simulink model "PD_Direct_Drive"  (R2016b)
settings: Solver=FixedStepAuto  StartTime=0.0  StopTime=inf  RelTol=1e-3  EnableMultiTasking=on
undefined symbols (not defined in the file): RGBLED_COLOR_ENUM, RGBLED_MODE_ENUM
libraries: pixhawk_slib_sensors_actuators x7, pixhawk_slib_misc_utils x6, simulink x2
settings Model: Creator=juanc  LastModifiedBy=pixhawk
settings OptimizationCC: DefaultParameterBehavior=Inlined  InlineInvariantSignals=on  LifeSpan=1  MaxStackSize=64
settings DebuggingCC: SFUnexpectedBacktrackingDiag=warning  SFNoUnconditionalDefaultTransitionDiag=warning  SFExecutionAtInitializationDiag=none
settings HardwareCC: ProdBitPerPointer=32  ProdBitPerSizeT=32  ProdBitPerPtrDiffT=32  ProdLargestAtomicInteger=Long  ProdLargestAtomicFloat=Double  ProdWordSize=32  ProdHWDeviceType=ARM Compatible->ARM Cortex
settings RTWCC: SystemTargetFile=ert.tlc  HardwareBoard=Pixhawk PX4  TLCOptions=-aInlineSetEventsForThisBaseRateFcn=TLC_FALSE -aSuppressMultiTaskScheduler=TLC_FALSE -aRateBasedStepFcn=0  TemplateMakefile=ert_default_tmf  Description=Embedded Coder  GenerateReport=on  Toolchain=Pixhawk Toolchain  IncludeHyperlinkInReport=on  LaunchReport=on  GenerateTraceInfo=on  GenerateTraceReport=on  GenerateTraceReportSl=on  GenerateTraceReportSf=on  GenerateTraceReportEml=on
settings CodeAppCC: ForceParamTrailComments=on  IgnoreCustomStorageClasses=off  OperatorAnnotations=on  SimulinkDataObjDesc=on  SFDataObjDesc=on  MATLABFcnDesc=on  InsertBlockDesc=on  MATLABSourceComments=on
settings ERTTargetCC: InlinedParameterPlacement=NonHierarchical  ERTCustomFileTemplate=PX4_codertarget_file_process.tlc
settings ConfigComp: CovMetricSettings=dw  CovHtmlReporting=on  CovSaveCumulativeToWorkspaceVar=on  CovSaveSingleToWorkspaceVar=on  CovExternalEMLEnable=off

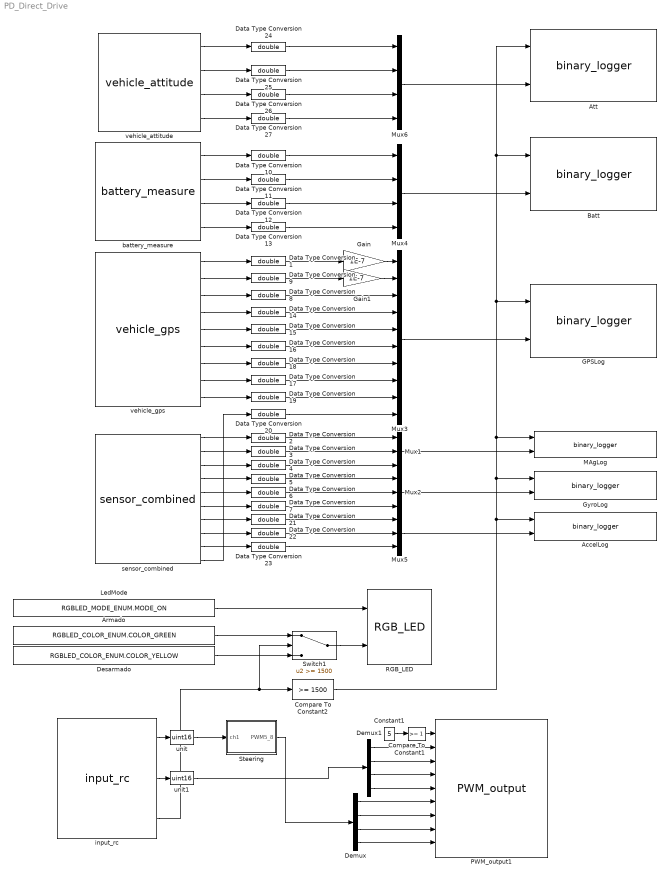
== system PD_Direct_Drive ==
  AccelLog : pixhawk_slib_misc_utils/binary_logger  logfile=/fs/microsd/log/acc  cacheflag=off  numRecs=1000
  Armado : Constant  Value=RGBLED_COLOR_ENUM.COLOR_GREEN  OutDataTypeStr=Enum: RGBLED_COLOR_ENUM
  Att : pixhawk_slib_misc_utils/binary_logger  logfile=/fs/microsd/log/att  cacheflag=off  numRecs=1000
  Batt : pixhawk_slib_misc_utils/binary_logger  logfile=/fs/microsd/log/bat  cacheflag=off  numRecs=1000
  Compare To Constant1 : simulink/Logic and Bit Operations/Compare To Constant  relop=>=  const=1  OutDataTypeStr=boolean
  Compare To Constant2 : simulink/Logic and Bit Operations/Compare To Constant  relop=>=  const=1500  OutDataTypeStr=boolean
  Constant1 : Constant  Value=5  OutDataTypeStr=Inherit: Inherit via back propagation  SampleTime=0.004
  Data Type Conversion{1..27} (27 alike) : DataTypeConversion  OutDataTypeStr=double
  Demux : Demux
  Demux1 : Demux
  Desarmado : Constant  Value=RGBLED_COLOR_ENUM.COLOR_YELLOW  OutDataTypeStr=Enum: RGBLED_COLOR_ENUM
  GPSLog : pixhawk_slib_misc_utils/binary_logger  logfile=/fs/microsd/log/GPS  cacheflag=off  numRecs=1000
  Gain : Gain  Gain=1E-7
  Gain1 : Gain  Gain=1E-7
  GyroLog : pixhawk_slib_misc_utils/binary_logger  logfile=/fs/microsd/log/gyr  cacheflag=off  numRecs=1000
  LedMode : Constant  Value=RGBLED_MODE_ENUM.MODE_ON  OutDataTypeStr=Enum: RGBLED_MODE_ENUM
  MAgLog : pixhawk_slib_misc_utils/binary_logger  logfile=/fs/microsd/log/mag  cacheflag=off  numRecs=1000
  Mux1 : Mux  Inputs=3
  Mux2 : Mux  Inputs=3
  Mux3 : Mux  Inputs=10
  Mux4 : Mux
  Mux5 : Mux  Inputs=3
  Mux6 : Mux
  PWM_output1 : pixhawk_slib_sensors_actuators/PWM_output  pwm_rate=50Hz  show_pwm1=on  show_pwm2=on  show_pwm3=on  show_pwm4=on  show_pwm5=on  show_pwm6=on  show_pwm7=on  show_pwm8=on
  RGB_LED : pixhawk_slib_sensors_actuators/RGB_LED
  Steering : MATLAB Function  TreatAsAtomicUnit=on
  Switch1 : Switch  Threshold=1500
  battery_measure : pixhawk_slib_sensors_actuators/battery_measure  SampleTime=1/250  VoltageOut=on  VoltageFilteredOut=off  CurrentOut=on  mAH_Out=on  TimeStamp=on
  input_rc : pixhawk_slib_sensors_actuators/input_rc  sampletime=1/250  channel1=on  channel2=off  channel3=on  channel4=off  channel5=off  channel6=off  channel7=on  channel8=off  ch_count=off  rssi=off  rc_failsafe=off  rc_lost=off  rc_inputsource=off
  sensor_combined : pixhawk_slib_sensors_actuators/sensor_combined  sampletime=1/250  show_mag=on  show_acc=on  show_gyro=on  show_baro=off  show_ts=on
  unit : DataTypeConversion  OutDataTypeStr=uint16
  unit1 : DataTypeConversion  OutDataTypeStr=uint16
  vehicle_attitude : pixhawk_slib_sensors_actuators/vehicle_attitude  sampletime=1/250  show_r=on  show_p=on  show_y=on  show_q=on
  vehicle_gps : pixhawk_slib_sensors_actuators/vehicle_gps  sampletime=1/250  show_ts_pos=on  show_alt=on  show_ts_gps=on  show_vel=on  show_fixtype=on  show_numsat=on
  wires:
  Switch1/1 -> RGB_LED/2
  Armado/1 -> Switch1/1
  Desarmado/1 -> Switch1/3
  LedMode/1 -> RGB_LED/1
  Data Type Conversion2/1 -> Mux1/1
  Data Type Conversion3/1 -> Mux1/2
  Data Type Conversion4/1 -> Mux1/3
  sensor_combined/2 -> Data Type Conversion3/1
  sensor_combined/3 -> Data Type Conversion4/1
  Mux2/1 -> GyroLog/2
  Data Type Conversion5/1 -> Mux2/1
  Data Type Conversion6/1 -> Mux2/2
  Data Type Conversion7/1 -> Mux2/3
  sensor_combined/1 -> Data Type Conversion2/1
  sensor_combined/4 -> Data Type Conversion5/1
  sensor_combined/5 -> Data Type Conversion6/1
  input_rc/3 -> Compare To Constant2/1, Switch1/2
  Mux3/1 -> GPSLog/2
  Compare To Constant2/1 -> Batt/1, Att/1, GPSLog/1, MAgLog/1, GyroLog/1, AccelLog/1
  Data Type Conversion1/1 -> Gain/1
  Data Type Conversion9/1 -> Gain1/1
  Data Type Conversion8/1 -> Mux3/3
  vehicle_gps/2 -> Data Type Conversion9/1
  vehicle_gps/3 -> Data Type Conversion8/1
  vehicle_gps/1 -> Data Type Conversion1/1
  vehicle_gps/4 -> Data Type Conversion14/1
  vehicle_gps/5 -> Data Type Conversion15/1
  vehicle_gps/9 -> Data Type Conversion19/1
  vehicle_gps/8 -> Data Type Conversion17/1
  vehicle_gps/7 -> Data Type Conversion18/1
  vehicle_gps/6 -> Data Type Conversion16/1
  battery_measure/4 -> Data Type Conversion13/1
  battery_measure/3 -> Data Type Conversion12/1
  battery_measure/1 -> Data Type Conversion10/1
  battery_measure/2 -> Data Type Conversion11/1
  Mux4/1 -> Batt/2
  Data Type Conversion10/1 -> Mux4/1
  Data Type Conversion11/1 -> Mux4/2
  Data Type Conversion12/1 -> Mux4/3
  Data Type Conversion14/1 -> Mux3/4
  Data Type Conversion15/1 -> Mux3/5
  Data Type Conversion13/1 -> Mux4/4
  Data Type Conversion16/1 -> Mux3/6
  Data Type Conversion17/1 -> Mux3/8
  Data Type Conversion18/1 -> Mux3/7
  Data Type Conversion19/1 -> Mux3/9
  Mux1/1 -> MAgLog/2
  Mux5/1 -> AccelLog/2
  Data Type Conversion21/1 -> Mux5/1
  Data Type Conversion22/1 -> Mux5/2
  Data Type Conversion23/1 -> Mux5/3
  sensor_combined/6 -> Data Type Conversion7/1
  sensor_combined/8 -> Data Type Conversion22/1
  sensor_combined/10 -> Data Type Conversion20/1
  Data Type Conversion20/1 -> Mux3/10
  vehicle_attitude/4 -> Data Type Conversion27/1
  vehicle_attitude/3 -> Data Type Conversion26/1
  vehicle_attitude/1 -> Data Type Conversion24/1
  vehicle_attitude/2 -> Data Type Conversion25/1
  Mux6/1 -> Att/2
  Data Type Conversion24/1 -> Mux6/1
  Data Type Conversion25/1 -> Mux6/2
  Data Type Conversion26/1 -> Mux6/3
  Data Type Conversion27/1 -> Mux6/4
  sensor_combined/7 -> Data Type Conversion21/1
  sensor_combined/9 -> Data Type Conversion23/1
  Gain/1 -> Mux3/1
  Gain1/1 -> Mux3/2
  Constant1/1 -> Compare To Constant1/1
  Compare To Constant1/1 -> PWM_output1/1
  input_rc/1 -> unit/1
  input_rc/2 -> unit1/1
  Demux/1 -> PWM_output1/6
  Demux/2 -> PWM_output1/7
  Demux/3 -> PWM_output1/8
  Demux/4 -> PWM_output1/9
  Steering/1(PWM5_8) -> Demux/1
  unit/1 -> Steering/1(ch1)
  Demux1/2 -> PWM_output1/3
  Demux1/3 -> PWM_output1/4
  Demux1/4 -> PWM_output1/5
  Demux1/1 -> PWM_output1/2
  unit1/1 -> Demux1/1

== matlab function PD_Direct_Drive/Steering ==
  data: ch1 input; PWM5_8 output
function PWM5_8 = fcn(ch1)
ang = uint16(((ch1-1500)*0.1)+1500);
PWM5_8 = [ang ang ang ang];
